simulink subsystem "keepWhileInFOV"  (R2024b)
settings: Solver=VariableStepAuto  StartTime=0.0  StopTime=10.0  RelTol=1e-3
undefined symbols (not defined in the file): sensors
libraries: simulink x2
settings Model: Creator=ricca  LastModifiedBy=ricca

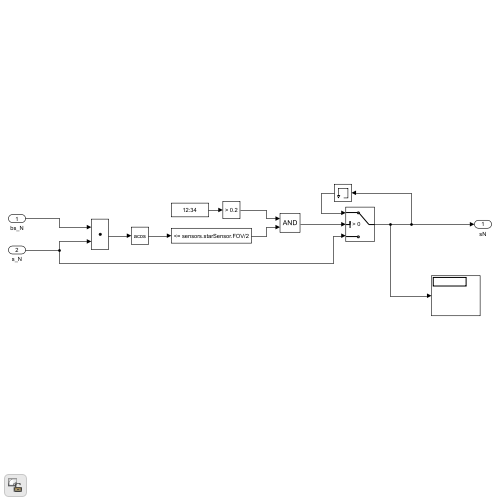
[thumbnail: Simulink's stored preview of the top-level diagram]
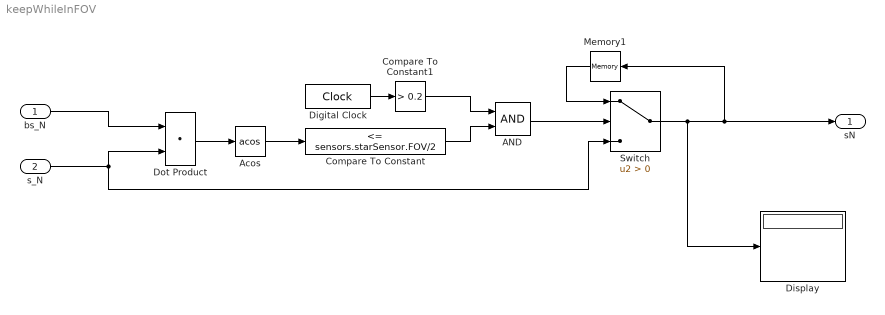
== system keepWhileInFOV ==
  bs_N : Inport
  s_N : Inport  Port=2
  AND : Logic  AllPortsSameDT=off  OutDataTypeStr=boolean
  Acos : Trigonometry  Operator=acos
  Compare To Constant : simulink/Logic and Bit Operations/Compare To Constant  relop=<=  const=sensors.starSensor.FOV/2  OutDataTypeStr=boolean
  Compare To Constant1 : simulink/Logic and Bit Operations/Compare To Constant  relop=>  const=0.2  OutDataTypeStr=boolean
  Digital Clock : DigitalClock  SampleTime=sensors.starSensor.sampleTime
  Display : Display
  Dot Product : DotProduct  OutDataTypeStr=Inherit: Inherit via internal rule
  Memory1 : Memory  InheritSampleTime=on
  Switch : Switch  Criteria=u2 > Threshold  SaturateOnIntegerOverflow=off  InputSameDT=off
  sN : Outport
  wires:
  Switch/1 -> Display/1, sN/1, Memory1/1
  s_N/1 -> Dot Product/2, Switch/3
  bs_N/1 -> Dot Product/1
  Dot Product/1 -> Acos/1
  Acos/1 -> Compare To Constant/1
  Memory1/1 -> Switch/1
  AND/1 -> Switch/2
  Digital Clock/1 -> Compare To Constant1/1
  Compare To Constant/1 -> AND/2
  Compare To Constant1/1 -> AND/1
